simulink model "aufgabe1_linear_reibung_c10_anfangsbedingung1"  (R2023b)
settings: Solver=VariableStepAuto  StartTime=0.0  StopTime=10.0  RelTol=1e-3
settings Model: Creator=serkan  LastModifiedBy=serkan

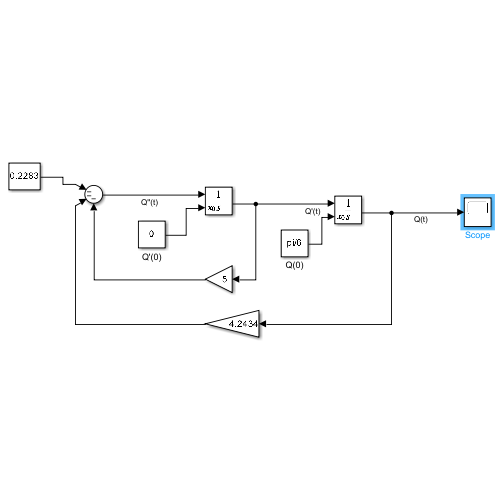
[thumbnail: Simulink's stored preview of the top-level diagram]
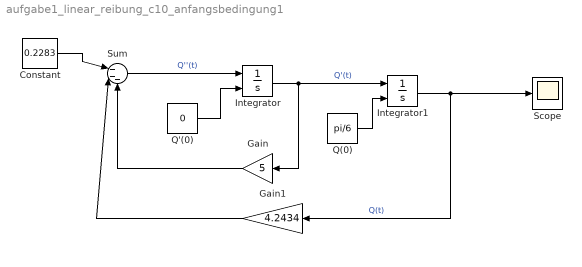
== system aufgabe1_linear_reibung_c10_anfangsbedingung1 ==
  Constant : Constant  Value=0.2283
  Gain : Gain  Gain=5
  Gain1 : Gain  Gain=4.2434
  Integrator : Integrator  InitialConditionSource=external
  Integrator1 : Integrator  InitialConditionSource=external
  Q'(0) : Constant  Value=0
  Q(0) : Constant  Value=pi/6
  Scope : Scope
  Sum : Sum  Inputs=|---
  wires:
  Gain1/1 -> Sum/2
  Constant/1 -> Sum/1
  Q'(0)/1 -> Integrator/2
  Q(0)/1 -> Integrator1/2
  Integrator1/1 -> Scope/1, Gain1/1  "Q(t)"
  Integrator/1 -> Integrator1/1, Gain/1  "Q'(t)"
  Gain/1 -> Sum/3
  Sum/1 -> Integrator/1  "Q''(t)"
